simulink model "wrist_flexion"  (Simulink 7.0)
settings: Solver=ode3  SolverMode=SingleTasking  StartTime=0.0  StopTime=Inf  FixedStep=.001  RelTol=1e-3
libraries: xpclib x5, xpcnilib x3, simulink x2, limblab x1
settings Model: Creator=Selket  LastModifiedBy=Christian  ExtModeArmWhenConnect=off  BufferReuse=off
settings OptimizationCC: BlockReduction=off  OptimizeBlockIOStorage=off  BufferReuse=off  ExpressionFolding=off  FoldNonRolledExpr=off  LocalBlockOutputs=off
settings DebuggingCC: SaveWithParameterizedLinksMsg=none  MultiTaskCondExecSysMsg=none  StrictBusMsg=None
settings RTWCC: SystemTargetFile=xpctarget.tlc  TemplateMakefile=xpc_default_tmf  Description=xPC Target  ProcessScript=xpctarget_make_rtw_hook  IncludeERTFirstTime=on
settings xpcTargetCC: TargetFcnLib=ansi_tfl_tmw.mat  GenFloatMathFcnCalls=ANSI_C  CompOptLevelCompliant=off  PortableWordSizes=off  xPCisDownloadable=off  xPCisDefaultEnv=off

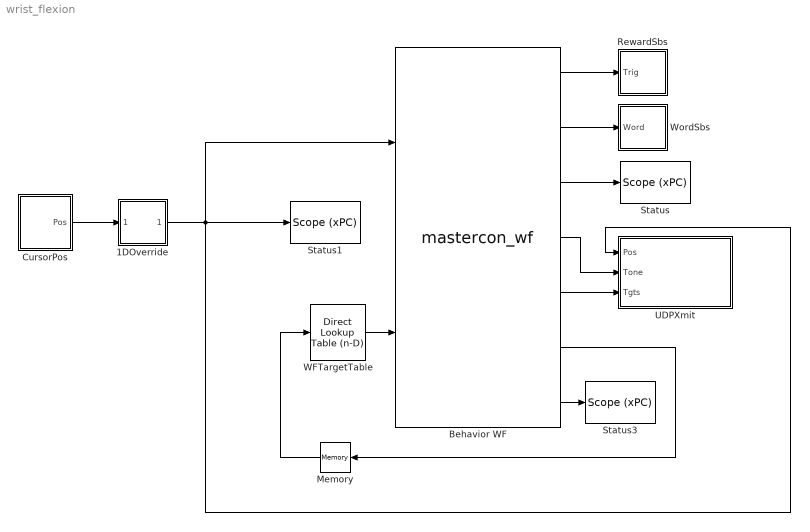
== system wrist_flexion ==
  1DOverride : Subsystem
  Behavior WF : S-Function  FunctionName=mastercon_wf  Parameters=8 5 .5 .5 1 2 2 2 2 2 0 0 0 0
      mask Display:
      | disp('Master Control\nWrist-Flexion')
      | port_label('input',1,'cursor')
      | port_label('input',2,'target list')
      | port_label('output',1,'Reward')
      | port_label('output',2,'Word')
      | port_label('output',3,'Status')
      | port_label('output',4,'Tone')
      | port_label('output',5,'Targets')
      | port_label('output',6,'Target Select')
      | port_label('output',7,'MVC Target')
  CursorPos : Subsystem
  Memory : Memory  Orientation=left  InheritSampleTime=on
  RewardSbs : Subsystem
  Status : xpclib/Misc./Scope (xPC)   SystemSampleTime=-1  scopeno=1  scopetype=Target  autostart=on  viewmode=Numerical  formatstr='%6.0f State,%6.0f Rewards,%6.0f Aborts,%6.0f Failures'  grid=on  ylimits=[-10,10]  nosamples=10  noprepostsamples=0  interleave=10  triggermode=FreeRun  triggersignal=1  triggerlevel=0.0  triggerslope=Either  triggerscope=1  triggersample=0  filename=data.dat  mode=Lazy  writesize=512  autorestart=off
  Status1 : xpclib/Misc./Scope (xPC)   SystemSampleTime=-1  scopeno=2  scopetype=Target  autostart=on  viewmode=Numerical  formatstr=' %6.6f X, %6.6f Y'  grid=on  ylimits=[-10,10]  nosamples=10  noprepostsamples=0  interleave=10  triggermode=FreeRun  triggersignal=1  triggerlevel=0.0  triggerslope=Either  triggerscope=1  triggersample=0  filename=data.dat  mode=Lazy  writesize=512  autorestart=off
  Status3 : xpclib/Misc./Scope (xPC)   SystemSampleTime=-1  scopeno=6  scopetype=Target  autostart=on  viewmode=Numerical  formatstr=' %6.4f X quad 1 MVC,%6.4f Y quad 1 MVC,%6.4f X quad 2 MVC,%6.4f Y quad 2 MVC,%6.4f X quad 3 MVC,%6.4f Y quad 3 MVC,%6.4f X quad 4 MVC,%6.4f Y quad 4 MVC'  grid=on  ylimits=[-10,10]  nosamples=10  noprepostsamples=0  interleave=10  triggermode=FreeRun  triggersignal=1  triggerlevel=0.0  triggerslope=Either  triggerscope=1  triggersample=0  filename=data.dat  mode=Lazy  writesize=512  autorestart=off
  UDPXmit : Subsystem
  WFTargetTable : simulink/Lookup Tables/Direct Lookup Table (n-D)  maskTabDims=2  explicitNumDims=1  outDims=Column  tabIsInput=off  mxTable=[5 5 5 5 5 5 5 5 5 5 5 5 5 5 5 5;5 5 5 5 5 5 5 5 5 5 5 5 5 5 5 5;5 5 5 5 5 5 5 5 5 5 5 5 5 5 5 5;5 5 5 5 5 5 5 5 5 5 5 5 5 5 5 5;0 0 0 0 0 0 0 0 0 0 0 0 0 0 0 0;0 0 0 0 0 0 0 0 0 0 0 0 0 0 0 0]  clipFlag=Warning  samptime=-1
  WordSbs : Subsystem
  wires:
  Behavior WF/2 -> WordSbs/1(Word)
  Behavior WF/1 -> RewardSbs/1(Trig)
  Memory/1 -> WFTargetTable/1
  WFTargetTable/1 -> Behavior WF/2
  Behavior WF/3 -> Status/1
  Behavior WF/4 -> UDPXmit/2(Tone)
  Behavior WF/5 -> UDPXmit/3(Tgts)
  CursorPos/1(Pos) -> 1DOverride/1(Trig)
  1DOverride/1(Out1) -> Status1/1, Behavior WF/1, UDPXmit/1(Pos)
  Behavior WF/6 -> Memory/1
  Behavior WF/7 -> Status3/1

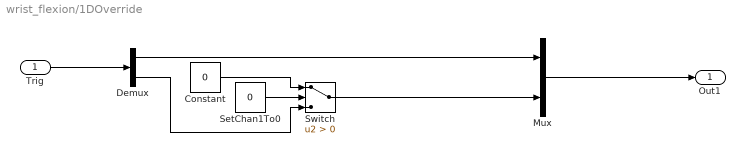
== system wrist_flexion/1DOverride ==
  Trig : Inport  OutDataType=sfix(16)  OutScaling=2^0
  Constant : Constant  Value=0  OutDataType=sfix(16)  OutScaling=2^0
  Demux : Demux  Outputs=2
  Mux : Mux  Inputs=2
  SetChan1To0 : Constant  Value=0  OutDataType=sfix(16)  OutScaling=2^0
  Switch : Switch  Criteria=u2 > Threshold
  Out1 : Outport  OutDataType=sfix(16)  OutScaling=2^0
  wires:
  Trig/1 -> Demux/1
  Switch/1 -> Mux/2
  Demux/1 -> Mux/1
  Mux/1 -> Out1/1
  SetChan1To0/1 -> Switch/2
  Constant/1 -> Switch/1
  Demux/2 -> Switch/3

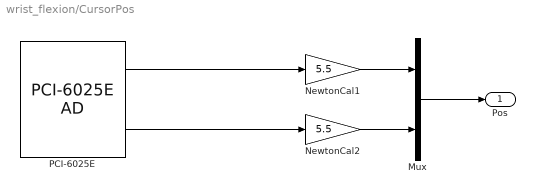
== system wrist_flexion/CursorPos ==
  Mux : Mux  Inputs=2
  NewtonCal1 : Gain  Gain=5.5  ParameterDataType=sfix(16)  ParameterScaling=2^0  OutDataType=sfix(16)  OutScaling=2^0
  NewtonCal2 : Gain  Gain=5.5  ParameterDataType=sfix(16)  ParameterScaling=2^0  OutDataType=sfix(16)  OutScaling=2^0
  "PCI-6025E " : xpcnilib/A//D/PCI-6025E AD  channel=[9 10]  range=[-10]  coupling=[0]  sampletime=0.001  slot=-1
  Pos : Outport  OutDataType=sfix(16)  OutScaling=2^0
  wires:
  "PCI-6025E "/1 -> NewtonCal1/1
  Mux/1 -> Pos/1
  NewtonCal1/1 -> Mux/1
  "PCI-6025E "/2 -> NewtonCal2/1
  NewtonCal2/1 -> Mux/2

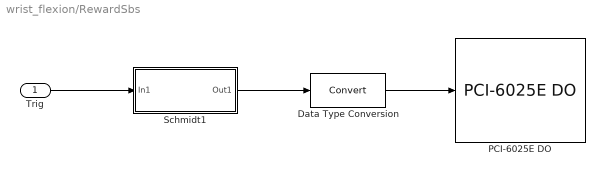
== system wrist_flexion/RewardSbs ==
  Trig : Inport  OutDataType=sfix(16)  OutScaling=2^0
  Data Type Conversion : DataTypeConversion  OutDataType=sfix(16)  OutScaling=2^0
  PCI-6025E DO : xpcnilib/Digital Output/PCI-6025E DO  channel=[2]  reset=[1]  initValue=[0]  sampletime=0.001  slot=-1
  Schmidt1 : Subsystem  mask(Schmidt Trigger){Time=.3}
      mask help: Creates an output pulse of the specified time in seconds when trig goes high
      mask Help: Creates an output pulse of the specified time in seconds when trig goes high
      mask Display:
      | port_label('output',1,'out')
      | port_label('input',1,'trig')
      | fprintf('t = %.2f',Time)
  wires:
  Trig/1 -> Schmidt1/1(In1)
  Data Type Conversion/1 -> PCI-6025E DO/1
  Schmidt1/1(Out1) -> Data Type Conversion/1

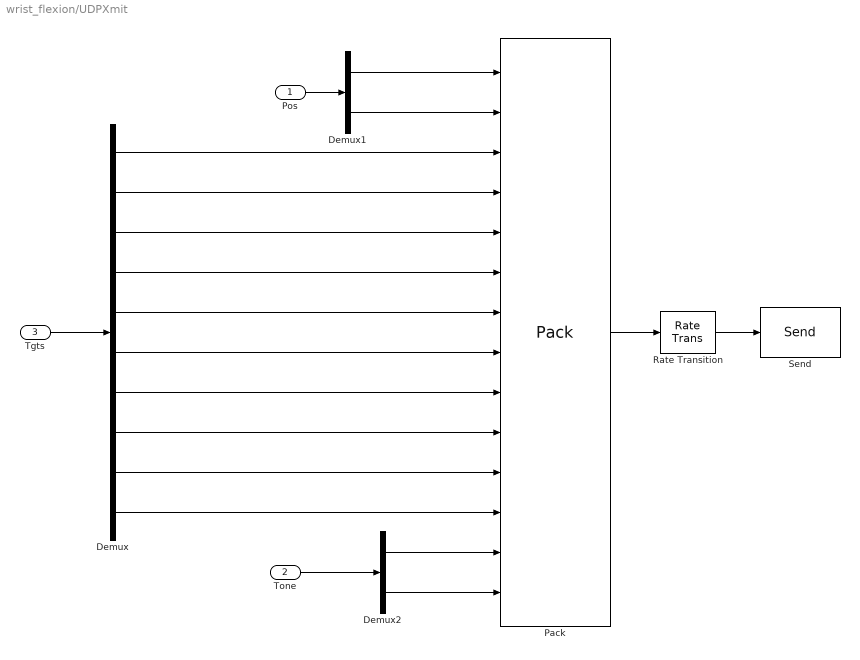
== system wrist_flexion/UDPXmit ==
  Pos : Inport  OutDataType=sfix(16)  OutScaling=2^0
  Tone : Inport  Port=2  OutDataType=sfix(16)  OutScaling=2^0
  Tgts : Inport  Port=3  OutDataType=sfix(16)  OutScaling=2^0
  Demux : Demux  Outputs=10
  Demux1 : Demux  Outputs=2
  Demux2 : Demux  Outputs=2
  Pack : xpclib/UDP/Pack  datatypes={'double', 'double','double','double','double','double','double','double','double','double','double','double','double','double'}  byteAlign=1
  Rate Transition : RateTransition
  Send : xpclib/UDP/Send  ipAddress=192.168.0.2  ipPort=25000  localPort=-1  sampletime=.02
  wires:
  Rate Transition/1 -> Send/1
  Pack/1 -> Rate Transition/1
  Demux/10 -> Pack/12
  Demux/9 -> Pack/11
  Demux/8 -> Pack/10
  Demux/7 -> Pack/9
  Demux/6 -> Pack/8
  Demux/5 -> Pack/7
  Demux/4 -> Pack/6
  Demux/3 -> Pack/5
  Demux/2 -> Pack/4
  Demux/1 -> Pack/3
  Demux1/1 -> Pack/1
  Demux1/2 -> Pack/2
  Pos/1 -> Demux1/1
  Demux2/1 -> Pack/13
  Demux2/2 -> Pack/14
  Tone/1 -> Demux2/1
  Tgts/1 -> Demux/1

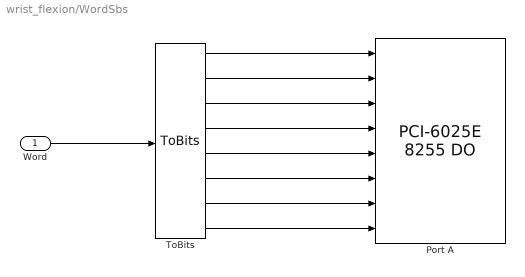
== system wrist_flexion/WordSbs ==
  Word : Inport  OutDataType=sfix(16)  OutScaling=2^0
  Port A : xpcnilib/Digital Output/PCI-6025E 8255 DO  channel=1:8  port=A  reset=[1]  initValue=[0]  chip=1  sampletime=-1  slot=[-1]
  ToBits : limblab/ToBits
  wires:
  Word/1 -> ToBits/1
  ToBits/1 -> Port A/1
  ToBits/2 -> Port A/2
  ToBits/3 -> Port A/3
  ToBits/4 -> Port A/4
  ToBits/5 -> Port A/5
  ToBits/6 -> Port A/6
  ToBits/7 -> Port A/7
  ToBits/8 -> Port A/8

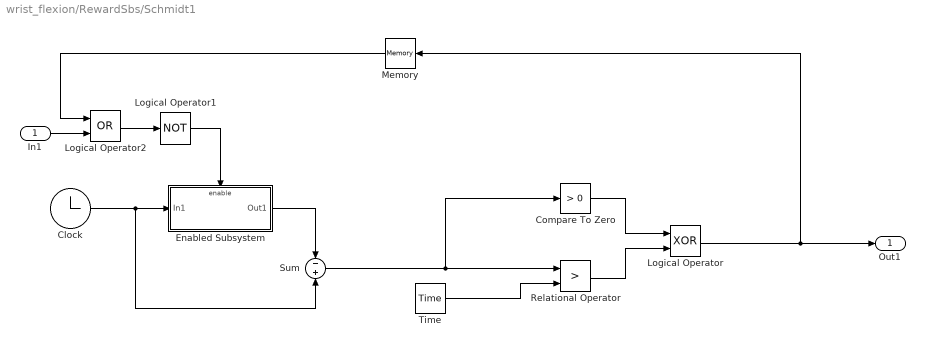
== system wrist_flexion/RewardSbs/Schmidt1 ==
  In1 : Inport  OutDataType=sfix(16)  OutScaling=2^0
  Clock : Clock
  Compare To Zero : simulink/Logic and Bit Operations/Compare To Zero  SystemSampleTime=-1  relop=>  LogicOutDataTypeMode=uint8  ZeroCross=off
  Enabled Subsystem : Subsystem  TreatAsAtomicUnit=on
  Logical Operator : Logic  Operator=XOR  AllPortsSameDT=off  OutDataTypeMode=boolean  SampleTime=.001
  Logical Operator1 : Logic  Operator=NOT  AllPortsSameDT=off  OutDataTypeMode=boolean
  Logical Operator2 : Logic  Operator=OR  AllPortsSameDT=off  OutDataTypeMode=boolean  SampleTime=.001
  Memory : Memory  Orientation=left
  Relational Operator : RelationalOperator  Operator=>  LogicOutDataTypeMode=boolean
  Sum : Sum  Inputs=-+  OutDataType=sfix(16)  OutScaling=2^0
  Time : Constant  Value=Time  OutDataType=sfix(16)  OutScaling=2^0
  Out1 : Outport  OutDataType=sfix(16)  OutScaling=2^0
  wires:
  Clock/1 -> Enabled Subsystem/1(In1), Sum/2
  Enabled Subsystem/1(Out1) -> Sum/1
  Sum/1 -> Compare To Zero/1, Relational Operator/1
  Time/1 -> Relational Operator/2
  Compare To Zero/1 -> Logical Operator/1
  Relational Operator/1 -> Logical Operator/2
  Logical Operator1/1 -> Enabled Subsystem/Enable
  Logical Operator/1 -> Out1/1, Memory/1
  In1/1 -> Logical Operator2/2
  Logical Operator2/1 -> Logical Operator1/1
  Memory/1 -> Logical Operator2/1

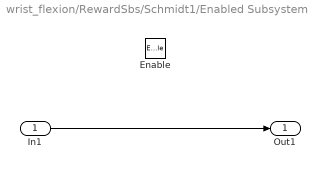
== system wrist_flexion/RewardSbs/Schmidt1/Enabled Subsystem ==
  In1 : Inport  OutDataType=sfix(16)  OutScaling=2^0
  Enable : EnablePort
  Out1 : Outport  OutDataType=sfix(16)  OutScaling=2^0
  wires:
  In1/1 -> Out1/1
